simulink subsystem "BUF_MIN_MAX_AVG"  (R2024a)
settings: Solver=VariableStepAuto  StartTime=0.0  StopTime=10.0  RelTol=1e-3
libraries: hdlsllib x1
settings Model: Creator=Jan Rosa  LastModifiedBy=Jan Rosa

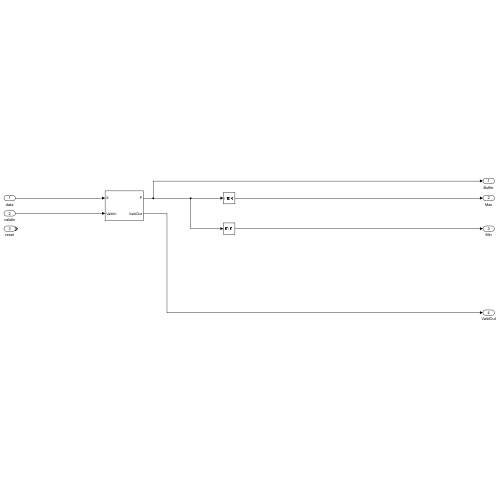
[thumbnail: Simulink's stored preview of the top-level diagram]
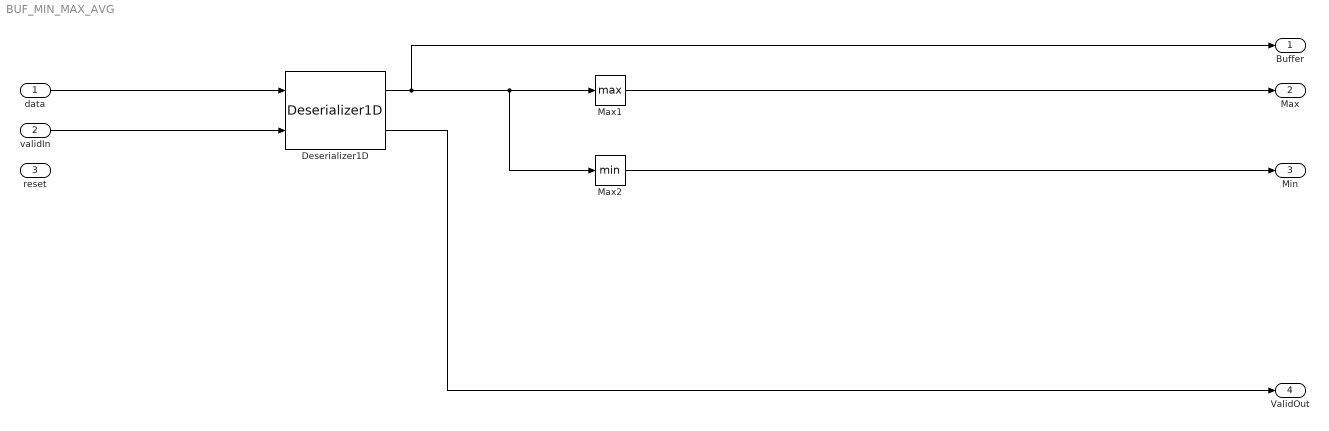
== system BUF_MIN_MAX_AVG ==
  data : Inport
  validIn : Inport  Port=2
  reset : Inport  Port=3
  Deserializer1D : hdlsllib/HDL Operations/Deserializer1D  Ratio=BUFFER_LEN  IdleCycles=0  InitialCondition=0  startIn=off  validIn=on  validOut=on  inputDataDimensions=-1  inputSampleTime=-1  inputSignalType=auto
  Max1 : MinMax  Function=max
  Max2 : MinMax
  Buffer : Outport
  Max : Outport  Port=2
  Min : Outport  Port=3
  ValidOut : Outport  Port=4
  wires:
  Deserializer1D/1 -> Max1/1, Max2/1, Buffer/1
  Max2/1 -> Min/1
  Deserializer1D/2 -> ValidOut/1
  validIn/1 -> Deserializer1D/2
  Max1/1 -> Max/1
  data/1 -> Deserializer1D/1
